simulink model "digital_control_4_2_2"  (R2021b)
settings: Solver=VariableStepAuto  StartTime=0.0  StopTime=10.0  RelTol=1e-3
values from neighbouring files (symbols this model uses):
  alpha = 10    [in_lab.m]
  f1 = F(1)    [in_lab.m]
  f2 = F(2)    [in_lab.m]
  T = 0.05    [in_lab.m]
  u_bar = sqrt(g*x_bar(1)^2)    [in_lab.m]    (also in prelab.m)
  x_bar = [0.5; 0.0]    [in_lab.m]    (also in prelab.m)
libraries: cstblocks x1
settings Model: Creator=pranshumalik14  LastModifiedBy=varunsampat
settings SolverCC: AlgebraicLoopSolver=TrustRegion
settings DataIOCC: ReturnWorkspaceOutputs=off
settings DebuggingCC: SFMachineParentedDataDiag=warning  ArithmeticOperatorsInVariantConditions=warning
settings SFSimCC: CustomCodeUndefinedFunction=UseInterfaceOnly

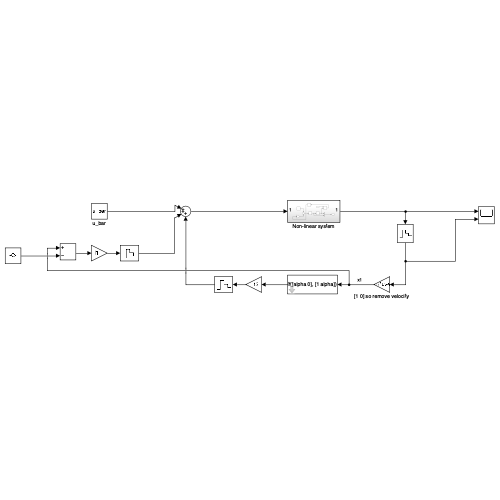
[thumbnail: Simulink's stored preview of the top-level diagram]
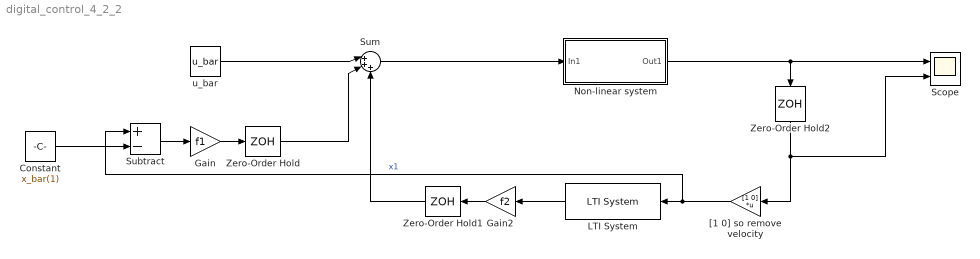
== system digital_control_4_2_2 ==
  Constant : Constant  Value=x_bar(1)
  Gain : Gain  Gain=f1
  Gain2 : Gain  Gain=f2
  LTI System : cstblocks/LTI System  sys=tf([alpha 0], [1 alpha])  IC=[]
  Non-linear system : Subsystem
  Scope : Scope  NumInputPorts=2
  Subtract : Sum  Inputs=+-
  Sum : Sum  Inputs=|+++
  Zero-Order Hold : ZeroOrderHold  SampleTime=T
  Zero-Order Hold1 : ZeroOrderHold  SampleTime=T
  Zero-Order Hold2 : ZeroOrderHold  SampleTime=T
  "[1 0] so remove velocity" : Gain  Gain=[1 0]  Multiplication=Matrix(K*u) (u vector)
  u_bar : Constant  Value=u_bar
  wires:
  Non-linear system/1(Out1) -> Zero-Order Hold2/1, Scope/1
  u_bar/1 -> Sum/1
  Sum/1 -> Non-linear system/1(In1)
  "[1 0] so remove velocity"/1 -> LTI System/1, Subtract/1  "x1"
  LTI System/1 -> Gain2/1
  Constant/1 -> Subtract/2
  Subtract/1 -> Gain/1
  Gain/1 -> Zero-Order Hold/1
  Zero-Order Hold/1 -> Sum/2
  Gain2/1 -> Zero-Order Hold1/1
  Zero-Order Hold1/1 -> Sum/3
  Zero-Order Hold2/1 -> Scope/2, "[1 0] so remove velocity"/1

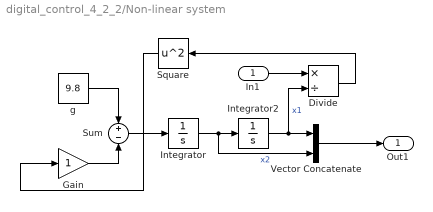
== system digital_control_4_2_2/Non-linear system ==
  In1 : Inport
  Divide : Product  Inputs=*/
  Gain : Gain
  Integrator : Integrator  InitialCondition=0.5
  Integrator2 : Integrator  InitialCondition=1.3
  Square : Math  Operator=square  SignedPower=on  SaturateOnIntegerOverflow=on
  Sum : Sum  Inputs=+-
  Vector Concatenate : Concatenate
  g : Constant  Value=9.8
  Out1 : Outport  VectorParamsAs1DForOutWhenUnconnected=off
  wires:
  Integrator2/1 -> Vector Concatenate/1, Divide/2  "x1"
  In1/1 -> Divide/1
  g/1 -> Sum/1
  Integrator/1 -> Vector Concatenate/2, Integrator2/1  "x2"
  Square/1 -> Gain/1
  Gain/1 -> Sum/2
  Sum/1 -> Integrator/1
  Divide/1 -> Square/1
  Vector Concatenate/1 -> Out1/1
